simulink model "STACK_Test"  (R2022a)
settings: Solver=FixedStepDiscrete  StartTime=0.0  StopTime=10.0  FixedStep=0.01  RelTol=1e-3
settings Model: Creator=User  LastModifiedBy=User

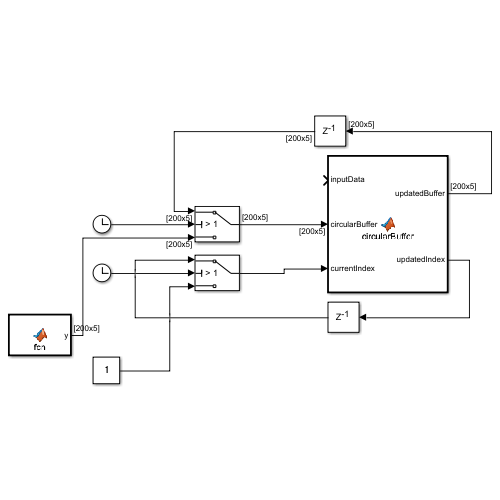
[thumbnail: Simulink's stored preview of the top-level diagram]
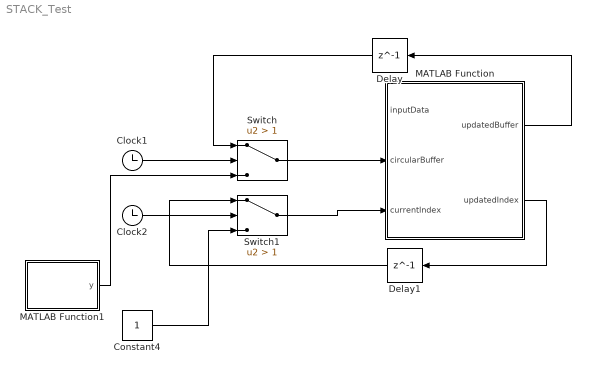
== system STACK_Test ==
  Clock1 : Clock
  Clock2 : Clock
  Constant4 : Constant
  Delay : Delay  DelayLength=1
  Delay1 : Delay  DelayLength=1
  MATLAB Function : MATLAB Function  TreatAsAtomicUnit=on
  MATLAB Function1 : MATLAB Function  TreatAsAtomicUnit=on
  Switch : Switch  Criteria=u2 > Threshold  Threshold=1  SaturateOnIntegerOverflow=off  InputSameDT=off
  Switch1 : Switch  Criteria=u2 > Threshold  Threshold=1  SaturateOnIntegerOverflow=off  InputSameDT=off
  wires:
  Switch/1 -> MATLAB Function/2(circularBuffer)
  Switch1/1 -> MATLAB Function/3(currentIndex)
  MATLAB Function/2(updatedIndex) -> Delay1/1
  Clock1/1 -> Switch/2
  Clock2/1 -> Switch1/2
  Constant4/1 -> Switch1/3
  MATLAB Function1/1(y) -> Switch/3
  MATLAB Function/1(updatedBuffer) -> Delay/1
  Delay/1 -> Switch/1
  Delay1/1 -> Switch1/1

== matlab function STACK_Test/MATLAB Function1 ==
  data: y output
function y = fcn()

y = zeros(200,5);

== matlab function STACK_Test/MATLAB Function ==
  data: inputData input; updatedBuffer output; circularBuffer input; currentIndex input; updatedIndex output
function [updatedBuffer, updatedIndex] = circularBuffer(inputData, circularBuffer, currentIndex)
    updatedBuffer = zeros(200,5);
    % Update index
    if currentIndex ~= 200
        updatedIndex = currentIndex +1 ;
    else
        updatedIndex = currentIndex;
    end
    
    % Update circular buffer
    updatedBuffer(1:currentIndex-1,:) = circularBuffer(2:currentIndex,:);
    updatedBuffer(currentIndex, :) = inputData;
    

end
